simulink model "Cooperative_Localization_05_New"  (R2016b)
settings: Solver=ode45  StartTime=0.0  StopTime=200  RelTol=1e-3  EnableMultiTasking=on
InitFcn:
  | Const_Coop_Local_05
values from neighbouring files (symbols this model uses):
  k1 = 1    [Const_05.m]
  k2 = 1    [Const_05.m]
undefined symbols (not defined in the file or in its folder): alpha, AN, B, B_pseudo_inverse, BBT_inv, BN, D, Delta_form, Gama0, gamma0, gamma_0, gamma_1, H, K, KI, Ki_1, Ki_2, Ki_3, Ki_4, lambda, m_cont, Mb, Mu, n, N, n_cont, Observer_Gain, P_struct, Q, Q1, R, Rho1, Rho_0, rho_0, rho_1, t_cont, U_dot0_M
(part 2 of 3)

== system Cooperative_Localization_05_New/Agent-2/Cooperative controller-2/Decenteralized Cooperaive Controller #2/Estimator A#2/Estimation Error ==
  X : Inport
  U : Inport  Port=2
  G_hat : Inport  Port=3
  Constant : Constant  Value=B
  Constant1 : Constant  Value=D
  Product : Product  Multiplication=Matrix(*)
  Product1 : Product  Multiplication=Matrix(*)
  Scope{1..5} (5 alike) : Scope
  Subsystem : Subsystem
  Subsystem1 : Subsystem
  Subsystem2 : Subsystem
  Subsystem3 : Subsystem
  Sum : Sum  Inputs=+--
  r : Outport
  wt : Outport  Port=2
  wires:
  G_hat/1 -> Product1/2
  Subsystem3/1(X_f) -> r/1, Scope4/1
  X/1 -> Subsystem/1(X), Subsystem3/1(X)
  Subsystem2/1(G_hatf) -> Sum/3, Scope2/1
  Subsystem1/1(Uf) -> Scope1/1, Sum/2
  Subsystem/1(Xf) -> Sum/1, Scope5/1
  Product1/1 -> Subsystem2/1(G_hat)
  Product/1 -> Subsystem1/1(U)
  Constant1/1 -> Product1/1
  U/1 -> Product/2
  Constant/1 -> Product/1
  Sum/1 -> wt/1, Scope3/1

== system Cooperative_Localization_05_New/Agent-2/Cooperative controller-2/Decenteralized Cooperaive Controller #2/Estimator A#2/For matrix Plot1 ==
  A : Inport
  MATLAB Function : MATLAB Function  TreatAsAtomicUnit=on
  To Workspace : ToWorkspace  VariableName=A_hat_2  SaveFormat=Structure With Time  SampleTime=-1
  wires:
  MATLAB Function/1(y) -> To Workspace/1
  A/1 -> MATLAB Function/1(u)

== system Cooperative_Localization_05_New/Agent-2/Cooperative controller-2/Decenteralized Cooperaive Controller #2/Estimator A#2/For matrix Plot2 ==
  A_dot : Inport
  MATLAB Function : MATLAB Function  TreatAsAtomicUnit=on
  To Workspace : ToWorkspace  VariableName=DA_hat_2  SaveFormat=Structure With Time  SampleTime=-1
  wires:
  A_dot/1 -> MATLAB Function/1(u)
  MATLAB Function/1(y) -> To Workspace/1

== system Cooperative_Localization_05_New/Agent-3/Cooperative controller-3/Decenteralized Cooperaive Controller #3/Estimator A#3/Estimation Error ==
  X : Inport
  U : Inport  Port=2
  G_hat : Inport  Port=3
  Constant : Constant  Value=B
  Constant1 : Constant  Value=D
  Product : Product  Multiplication=Matrix(*)
  Product1 : Product  Multiplication=Matrix(*)
  Scope{1..5} (5 alike) : Scope
  Subsystem : Subsystem
  Subsystem1 : Subsystem
  Subsystem2 : Subsystem
  Subsystem3 : Subsystem
  Sum : Sum  Inputs=+--
  r : Outport
  wt : Outport  Port=2
  wires:
  G_hat/1 -> Product1/2
  Subsystem3/1(X_f) -> r/1, Scope4/1
  X/1 -> Subsystem/1(X), Subsystem3/1(X)
  Subsystem2/1(G_hatf) -> Sum/3, Scope2/1
  Subsystem1/1(Uf) -> Scope1/1, Sum/2
  Subsystem/1(Xf) -> Sum/1, Scope5/1
  Product1/1 -> Subsystem2/1(G_hat)
  Product/1 -> Subsystem1/1(U)
  Constant1/1 -> Product1/1
  U/1 -> Product/2
  Constant/1 -> Product/1
  Sum/1 -> wt/1, Scope3/1

== system Cooperative_Localization_05_New/Agent-3/Cooperative controller-3/Decenteralized Cooperaive Controller #3/Estimator A#3/For matrix Plot1 ==
  A : Inport
  MATLAB Function : MATLAB Function  TreatAsAtomicUnit=on
  To Workspace : ToWorkspace  VariableName=A_hat_3  SaveFormat=Structure With Time  SampleTime=-1
  wires:
  MATLAB Function/1(y) -> To Workspace/1
  A/1 -> MATLAB Function/1(u)

== system Cooperative_Localization_05_New/Agent-3/Cooperative controller-3/Decenteralized Cooperaive Controller #3/Estimator A#3/For matrix Plot2 ==
  A_dot : Inport
  MATLAB Function : MATLAB Function  TreatAsAtomicUnit=on
  To Workspace : ToWorkspace  VariableName=DA_hat_3  SaveFormat=Structure With Time  SampleTime=-1
  wires:
  A_dot/1 -> MATLAB Function/1(u)
  MATLAB Function/1(y) -> To Workspace/1

== system Cooperative_Localization_05_New/Agent-4/Cooperative controller-4/Decenteralized Cooperaive Controller #4/Estimator A#4/Estimation Error ==
  X : Inport
  U : Inport  Port=2
  G_hat : Inport  Port=3
  Constant : Constant  Value=B
  Constant1 : Constant  Value=D
  Product : Product  Multiplication=Matrix(*)
  Product1 : Product  Multiplication=Matrix(*)
  Scope{1..5} (5 alike) : Scope
  Subsystem : Subsystem
  Subsystem1 : Subsystem
  Subsystem2 : Subsystem
  Subsystem3 : Subsystem
  Sum : Sum  Inputs=+--
  r : Outport
  wt : Outport  Port=2
  wires:
  G_hat/1 -> Product1/2
  Subsystem3/1(X_f) -> r/1, Scope4/1
  X/1 -> Subsystem/1(X), Subsystem3/1(X)
  Subsystem2/1(G_hatf) -> Sum/3, Scope2/1
  Subsystem1/1(Uf) -> Scope1/1, Sum/2
  Subsystem/1(Xf) -> Sum/1, Scope5/1
  Product1/1 -> Subsystem2/1(G_hat)
  Product/1 -> Subsystem1/1(U)
  Constant1/1 -> Product1/1
  U/1 -> Product/2
  Constant/1 -> Product/1
  Sum/1 -> wt/1, Scope3/1

== system Cooperative_Localization_05_New/Agent-4/Cooperative controller-4/Decenteralized Cooperaive Controller #4/Estimator A#4/For matrix Plot1 ==
  A : Inport
  MATLAB Function : MATLAB Function  TreatAsAtomicUnit=on
  To Workspace : ToWorkspace  VariableName=A_hat_4  SaveFormat=Structure With Time  SampleTime=-1
  wires:
  MATLAB Function/1(y) -> To Workspace/1
  A/1 -> MATLAB Function/1(u)

== system Cooperative_Localization_05_New/Agent-4/Cooperative controller-4/Decenteralized Cooperaive Controller #4/Estimator A#4/For matrix Plot2 ==
  A_dot : Inport
  MATLAB Function : MATLAB Function  TreatAsAtomicUnit=on
  To Workspace : ToWorkspace  VariableName=DA_hat_4  SaveFormat=Structure With Time  SampleTime=-1
  wires:
  A_dot/1 -> MATLAB Function/1(u)
  MATLAB Function/1(y) -> To Workspace/1

== system Cooperative_Localization_05_New/Agent-1/Cooperative controller-1/Decenteralized Cooperaive Controller #1/Estimator A#1/Estimation Error/Subsystem ==
  X : Inport
  Demux : Demux
  Mux : Mux
  Transfer Fcn{,1..3} (4 alike) : TransferFcn  Numerator=[1 0]  Denominator=[1 1]
  Xf : Outport
  wires:
  Demux/1 -> Transfer Fcn/1
  Transfer Fcn/1 -> Mux/1
  Mux/1 -> Xf/1
  X/1 -> Demux/1
  Demux/2 -> Transfer Fcn1/1
  Transfer Fcn1/1 -> Mux/2
  Demux/3 -> Transfer Fcn2/1
  Transfer Fcn2/1 -> Mux/3
  Transfer Fcn3/1 -> Mux/4
  Demux/4 -> Transfer Fcn3/1

== system Cooperative_Localization_05_New/Agent-1/Cooperative controller-1/Decenteralized Cooperaive Controller #1/Estimator A#1/Estimation Error/Subsystem1 ==
  U : Inport
  Demux : Demux
  Mux : Mux
  Transfer Fcn{1..4} (4 alike) : TransferFcn  Denominator=[1 1]
  Uf : Outport
  wires:
  U/1 -> Demux/1
  Mux/1 -> Uf/1
  Transfer Fcn1/1 -> Mux/1
  Demux/1 -> Transfer Fcn1/1
  Transfer Fcn2/1 -> Mux/2
  Demux/2 -> Transfer Fcn2/1
  Demux/3 -> Transfer Fcn3/1
  Transfer Fcn3/1 -> Mux/3
  Transfer Fcn4/1 -> Mux/4
  Demux/4 -> Transfer Fcn4/1

== system Cooperative_Localization_05_New/Agent-1/Cooperative controller-1/Decenteralized Cooperaive Controller #1/Estimator A#1/Estimation Error/Subsystem2 ==
  G_hat : Inport
  Demux : Demux
  Mux : Mux
  Transfer Fcn{1..4} (4 alike) : TransferFcn  Denominator=[1 1]
  G_hatf : Outport
  wires:
  Demux/1 -> Transfer Fcn2/1
  Transfer Fcn2/1 -> Mux/1
  Mux/1 -> G_hatf/1
  G_hat/1 -> Demux/1
  Demux/2 -> Transfer Fcn1/1
  Transfer Fcn1/1 -> Mux/2
  Demux/3 -> Transfer Fcn3/1
  Transfer Fcn3/1 -> Mux/3
  Demux/4 -> Transfer Fcn4/1
  Transfer Fcn4/1 -> Mux/4

== system Cooperative_Localization_05_New/Agent-1/Cooperative controller-1/Decenteralized Cooperaive Controller #1/Estimator A#1/Estimation Error/Subsystem3 ==
  X : Inport
  Demux : Demux
  Mux : Mux
  Transfer Fcn{1..4} (4 alike) : TransferFcn  Denominator=[1 1]
  X_f : Outport
  wires:
  X/1 -> Demux/1
  Mux/1 -> X_f/1
  Transfer Fcn2/1 -> Mux/1
  Demux/1 -> Transfer Fcn2/1
  Demux/2 -> Transfer Fcn1/1
  Transfer Fcn1/1 -> Mux/2
  Demux/3 -> Transfer Fcn3/1
  Transfer Fcn3/1 -> Mux/3
  Demux/4 -> Transfer Fcn4/1
  Transfer Fcn4/1 -> Mux/4

== system Cooperative_Localization_05_New/Agent-2/Cooperative controller-2/Decenteralized Cooperaive Controller #2/Estimator A#2/Estimation Error/Subsystem ==
  X : Inport
  Demux : Demux
  Mux : Mux
  Transfer Fcn{,1..3} (4 alike) : TransferFcn  Numerator=[1 0]  Denominator=[1 1]
  Xf : Outport
  wires:
  Demux/1 -> Transfer Fcn/1
  Transfer Fcn/1 -> Mux/1
  Mux/1 -> Xf/1
  X/1 -> Demux/1
  Demux/2 -> Transfer Fcn1/1
  Transfer Fcn1/1 -> Mux/2
  Demux/3 -> Transfer Fcn2/1
  Transfer Fcn2/1 -> Mux/3
  Transfer Fcn3/1 -> Mux/4
  Demux/4 -> Transfer Fcn3/1

== system Cooperative_Localization_05_New/Agent-2/Cooperative controller-2/Decenteralized Cooperaive Controller #2/Estimator A#2/Estimation Error/Subsystem1 ==
  U : Inport
  Demux : Demux
  Mux : Mux
  Transfer Fcn{1..4} (4 alike) : TransferFcn  Denominator=[1 1]
  Uf : Outport
  wires:
  U/1 -> Demux/1
  Mux/1 -> Uf/1
  Transfer Fcn1/1 -> Mux/1
  Demux/1 -> Transfer Fcn1/1
  Transfer Fcn2/1 -> Mux/2
  Demux/2 -> Transfer Fcn2/1
  Demux/3 -> Transfer Fcn3/1
  Transfer Fcn3/1 -> Mux/3
  Transfer Fcn4/1 -> Mux/4
  Demux/4 -> Transfer Fcn4/1

== system Cooperative_Localization_05_New/Agent-2/Cooperative controller-2/Decenteralized Cooperaive Controller #2/Estimator A#2/Estimation Error/Subsystem2 ==
  G_hat : Inport
  Demux : Demux
  Mux : Mux
  Transfer Fcn{1..4} (4 alike) : TransferFcn  Denominator=[1 1]
  G_hatf : Outport
  wires:
  Demux/1 -> Transfer Fcn2/1
  Transfer Fcn2/1 -> Mux/1
  Mux/1 -> G_hatf/1
  G_hat/1 -> Demux/1
  Demux/2 -> Transfer Fcn1/1
  Transfer Fcn1/1 -> Mux/2
  Demux/3 -> Transfer Fcn3/1
  Transfer Fcn3/1 -> Mux/3
  Demux/4 -> Transfer Fcn4/1
  Transfer Fcn4/1 -> Mux/4

== system Cooperative_Localization_05_New/Agent-2/Cooperative controller-2/Decenteralized Cooperaive Controller #2/Estimator A#2/Estimation Error/Subsystem3 ==
  X : Inport
  Demux : Demux
  Mux : Mux
  Transfer Fcn{1..4} (4 alike) : TransferFcn  Denominator=[1 1]
  X_f : Outport
  wires:
  X/1 -> Demux/1
  Mux/1 -> X_f/1
  Transfer Fcn2/1 -> Mux/1
  Demux/1 -> Transfer Fcn2/1
  Demux/2 -> Transfer Fcn1/1
  Transfer Fcn1/1 -> Mux/2
  Demux/3 -> Transfer Fcn3/1
  Transfer Fcn3/1 -> Mux/3
  Demux/4 -> Transfer Fcn4/1
  Transfer Fcn4/1 -> Mux/4

== system Cooperative_Localization_05_New/Agent-3/Cooperative controller-3/Decenteralized Cooperaive Controller #3/Estimator A#3/Estimation Error/Subsystem ==
  X : Inport
  Demux : Demux
  Mux : Mux
  Transfer Fcn{,1..3} (4 alike) : TransferFcn  Numerator=[1 0]  Denominator=[1 1]
  Xf : Outport
  wires:
  Demux/1 -> Transfer Fcn/1
  Transfer Fcn/1 -> Mux/1
  Mux/1 -> Xf/1
  X/1 -> Demux/1
  Demux/2 -> Transfer Fcn1/1
  Transfer Fcn1/1 -> Mux/2
  Demux/3 -> Transfer Fcn2/1
  Transfer Fcn2/1 -> Mux/3
  Transfer Fcn3/1 -> Mux/4
  Demux/4 -> Transfer Fcn3/1

== system Cooperative_Localization_05_New/Agent-3/Cooperative controller-3/Decenteralized Cooperaive Controller #3/Estimator A#3/Estimation Error/Subsystem1 ==
  U : Inport
  Demux : Demux
  Mux : Mux
  Transfer Fcn{1..4} (4 alike) : TransferFcn  Denominator=[1 1]
  Uf : Outport
  wires:
  U/1 -> Demux/1
  Mux/1 -> Uf/1
  Transfer Fcn1/1 -> Mux/1
  Demux/1 -> Transfer Fcn1/1
  Transfer Fcn2/1 -> Mux/2
  Demux/2 -> Transfer Fcn2/1
  Demux/3 -> Transfer Fcn3/1
  Transfer Fcn3/1 -> Mux/3
  Transfer Fcn4/1 -> Mux/4
  Demux/4 -> Transfer Fcn4/1

== system Cooperative_Localization_05_New/Agent-3/Cooperative controller-3/Decenteralized Cooperaive Controller #3/Estimator A#3/Estimation Error/Subsystem2 ==
  G_hat : Inport
  Demux : Demux
  Mux : Mux
  Transfer Fcn{1..4} (4 alike) : TransferFcn  Denominator=[1 1]
  G_hatf : Outport
  wires:
  Demux/1 -> Transfer Fcn2/1
  Transfer Fcn2/1 -> Mux/1
  Mux/1 -> G_hatf/1
  G_hat/1 -> Demux/1
  Demux/2 -> Transfer Fcn1/1
  Transfer Fcn1/1 -> Mux/2
  Demux/3 -> Transfer Fcn3/1
  Transfer Fcn3/1 -> Mux/3
  Demux/4 -> Transfer Fcn4/1
  Transfer Fcn4/1 -> Mux/4

== system Cooperative_Localization_05_New/Agent-3/Cooperative controller-3/Decenteralized Cooperaive Controller #3/Estimator A#3/Estimation Error/Subsystem3 ==
  X : Inport
  Demux : Demux
  Mux : Mux
  Transfer Fcn{1..4} (4 alike) : TransferFcn  Denominator=[1 1]
  X_f : Outport
  wires:
  X/1 -> Demux/1
  Mux/1 -> X_f/1
  Transfer Fcn2/1 -> Mux/1
  Demux/1 -> Transfer Fcn2/1
  Demux/2 -> Transfer Fcn1/1
  Transfer Fcn1/1 -> Mux/2
  Demux/3 -> Transfer Fcn3/1
  Transfer Fcn3/1 -> Mux/3
  Demux/4 -> Transfer Fcn4/1
  Transfer Fcn4/1 -> Mux/4

== system Cooperative_Localization_05_New/Agent-4/Cooperative controller-4/Decenteralized Cooperaive Controller #4/Estimator A#4/Estimation Error/Subsystem ==
  X : Inport
  Demux : Demux
  Mux : Mux
  Transfer Fcn{,1..3} (4 alike) : TransferFcn  Numerator=[1 0]  Denominator=[1 1]
  Xf : Outport
  wires:
  Demux/1 -> Transfer Fcn/1
  Transfer Fcn/1 -> Mux/1
  Mux/1 -> Xf/1
  X/1 -> Demux/1
  Demux/2 -> Transfer Fcn1/1
  Transfer Fcn1/1 -> Mux/2
  Demux/3 -> Transfer Fcn2/1
  Transfer Fcn2/1 -> Mux/3
  Transfer Fcn3/1 -> Mux/4
  Demux/4 -> Transfer Fcn3/1

== system Cooperative_Localization_05_New/Agent-4/Cooperative controller-4/Decenteralized Cooperaive Controller #4/Estimator A#4/Estimation Error/Subsystem1 ==
  U : Inport
  Demux : Demux
  Mux : Mux
  Transfer Fcn{1..4} (4 alike) : TransferFcn  Denominator=[1 1]
  Uf : Outport
  wires:
  U/1 -> Demux/1
  Mux/1 -> Uf/1
  Transfer Fcn1/1 -> Mux/1
  Demux/1 -> Transfer Fcn1/1
  Transfer Fcn2/1 -> Mux/2
  Demux/2 -> Transfer Fcn2/1
  Demux/3 -> Transfer Fcn3/1
  Transfer Fcn3/1 -> Mux/3
  Transfer Fcn4/1 -> Mux/4
  Demux/4 -> Transfer Fcn4/1

== system Cooperative_Localization_05_New/Agent-4/Cooperative controller-4/Decenteralized Cooperaive Controller #4/Estimator A#4/Estimation Error/Subsystem2 ==
  G_hat : Inport
  Demux : Demux
  Mux : Mux
  Transfer Fcn{1..4} (4 alike) : TransferFcn  Denominator=[1 1]
  G_hatf : Outport
  wires:
  Demux/1 -> Transfer Fcn2/1
  Transfer Fcn2/1 -> Mux/1
  Mux/1 -> G_hatf/1
  G_hat/1 -> Demux/1
  Demux/2 -> Transfer Fcn1/1
  Transfer Fcn1/1 -> Mux/2
  Demux/3 -> Transfer Fcn3/1
  Transfer Fcn3/1 -> Mux/3
  Demux/4 -> Transfer Fcn4/1
  Transfer Fcn4/1 -> Mux/4

== system Cooperative_Localization_05_New/Agent-4/Cooperative controller-4/Decenteralized Cooperaive Controller #4/Estimator A#4/Estimation Error/Subsystem3 ==
  X : Inport
  Demux : Demux
  Mux : Mux
  Transfer Fcn{1..4} (4 alike) : TransferFcn  Denominator=[1 1]
  X_f : Outport
  wires:
  X/1 -> Demux/1
  Mux/1 -> X_f/1
  Transfer Fcn2/1 -> Mux/1
  Demux/1 -> Transfer Fcn2/1
  Demux/2 -> Transfer Fcn1/1
  Transfer Fcn1/1 -> Mux/2
  Demux/3 -> Transfer Fcn3/1
  Transfer Fcn3/1 -> Mux/3
  Demux/4 -> Transfer Fcn4/1
  Transfer Fcn4/1 -> Mux/4

== matlab function Cooperative_Localization_05_New/Agent-1/Cooperative controller-1/Choosing real control variables ==
  data: u output; U input
function u = fcn(U)

u = U(3:4);

end

== matlab function Cooperative_Localization_05_New/Agent-1/Agent-1/MATLAB Function ==
  data: Px input; Py input; Vx input; out output; Vy input; Ax input; Ay input; t input
function out = fcn(Px,Py,Vx,Vy,Ax,Ay,t)

DPx = Vx;
DPy = Vy;

DVx = Ax - Vx * sin(0.2*t) + 0.5 * Px * cos(0.1*t);
DVy = Ay - Vy * sin(0.2*t) + 0.5 * Py * cos(0.1*t);

out = [DPx;DPy;DVx;DVy];

end

== matlab function Cooperative_Localization_05_New/Agent-2/Agent-2/MATLAB Function ==
  data: Px input; Py input; Vx input; out output; Vy input; Ax input; Ay input; t input
function out = fcn(Px,Py,Vx,Vy,Ax,Ay,t)

DPx = Vx;
DPy = Vy;

DVx = Ax - Vx * sin(0.2*t) + 0.5 * Px * cos(0.1*t);
DVy = Ay - Vy * sin(0.2*t) + 0.5 * Py * cos(0.1*t);

out = [DPx;DPy;DVx;DVy];

end

== matlab function Cooperative_Localization_05_New/Agent-2/Relative positions-2/Relative estimation ==
  data: V_rel input; d input; DP_est output; P_est input; alpha parameter
function DP_est = fcn(V_rel,d,P_est,alpha)

e = (d^2) - (P_est'*P_est);
g = P_est'*V_rel;

DP_est = (1 + alpha * sign(e*g)) * V_rel;

end

== matlab function Cooperative_Localization_05_New/Agent-2/Relative positions-2/Relative estimation1 ==
  data: V_rel input; d input; DP_est output; P_est input; alpha parameter
function DP_est = fcn(V_rel,d,P_est,alpha)

e = (d^2) - (P_est'*P_est);
g = P_est'*V_rel;

DP_est = (1 + alpha * sign(e*g)) * V_rel;

end

== matlab function Cooperative_Localization_05_New/Agent-2/Relative positions-2/Relative estimation2 ==
  data: V_rel input; d input; DP_est output; P_est input; alpha parameter
function DP_est = fcn(V_rel,d,P_est,alpha)

e = (d^2) - (P_est'*P_est);
g = P_est'*V_rel;

DP_est = (1 + alpha * sign(e*g)) * V_rel;

end

== matlab function Cooperative_Localization_05_New/Agent-2/Relative positions-2/Relative estimation3 ==
  data: V_rel input; d input; DP_est output; P_est input; alpha parameter
function DP_est = fcn(V_rel,d,P_est,alpha)

e = (d^2) - (P_est'*P_est);
g = P_est'*V_rel;

DP_est = (1 + alpha * sign(e*g)) * V_rel;

end

== matlab function Cooperative_Localization_05_New/Agent-1/observer-1 ==
  data: P_hat input; tau input; P0 input; P_rel_local input; P_rel0_local input; AN parameter; BN parameter; H parameter; DP_hat_local output; n parameter; N parameter; Num input; Mu parameter; Mb parameter; tau_i output; alpha parameter
function [DP_hat_local,tau_i] = fcn(P_hat,tau,P0,P_rel_local,P_rel0_local,AN,BN,H,n,N,Num,Mu,Mb,alpha)

P_hat_in = zeros(n,N);
P_rel_local_in = zeros(n,N);
tau_in = zeros(n,N);
for i=1:N
    P_hat_in(:,i) = P_hat((i-1)*n+1:(i*n),1); 
    P_rel_local_in(:,i) = P_rel_local((i-1)*n+1:(i*n),1); 
    tau_in(:,i) = tau((i-1)*n+1:(i*n),1);
end

e = BN(Num,Num)*(P_hat_in(:,Num) - (P0 + P_rel0_local));
Vec = zeros(n,1);
for i=1:N
    e = e + ( AN(Num,i)*(P_hat_in(:,Num) - (P_hat_in(:,i) + P_rel_local_in(:,i))) ); 
    Vec = Vec + ( H(Num,i)*tau_in(:,i) );    
end

SGN_vec = Vec./(abs(Vec)+alpha);
SGN = diag(SGN_vec);    

DP_hat_local = - ( Mu*e ) - ( SGN*Mb );
tau_i = e;

end

== matlab function Cooperative_Localization_05_New/Agent-3/Relative positions-3/Relative estimation ==
  data: V_rel input; d input; DP_est output; P_est input; alpha parameter
function DP_est = fcn(V_rel,d,P_est,alpha)

e = (d^2) - (P_est'*P_est);
g = P_est'*V_rel;

DP_est = (1 + alpha * sign(e*g)) * V_rel;

end

== matlab function Cooperative_Localization_05_New/Agent-1/Relative positions-1/Relative estimation2 ==
  data: V_rel input; d input; DP_est output; P_est input; alpha parameter
function DP_est = fcn(V_rel,d,P_est,alpha)

e = (d^2) - (P_est'*P_est);
g = P_est'*V_rel;

DP_est = (1 + alpha * sign(e*g)) * V_rel;

end

== matlab function Cooperative_Localization_05_New/Agent-3/Relative positions-3/Relative estimation2 ==
  data: V_rel input; d input; DP_est output; P_est input; alpha parameter
function DP_est = fcn(V_rel,d,P_est,alpha)

e = (d^2) - (P_est'*P_est);
g = P_est'*V_rel;

DP_est = (1 + alpha * sign(e*g)) * V_rel;

end

== matlab function Cooperative_Localization_05_New/Agent-3/Relative positions-3/Relative estimation1 ==
  data: V_rel input; d input; DP_est output; P_est input; alpha parameter
function DP_est = fcn(V_rel,d,P_est,alpha)

e = (d^2) - (P_est'*P_est);
g = P_est'*V_rel;

DP_est = (1 + alpha * sign(e*g)) * V_rel;

end

== matlab function Cooperative_Localization_05_New/Agent-3/Relative positions-3/Relative estimation3 ==
  data: V_rel input; d input; DP_est output; P_est input; alpha parameter
function DP_est = fcn(V_rel,d,P_est,alpha)

e = (d^2) - (P_est'*P_est);
g = P_est'*V_rel;

DP_est = (1 + alpha * sign(e*g)) * V_rel;

end

== matlab function Cooperative_Localization_05_New/Agent-1/Cooperative controller-1/Decenteralized Cooperaive Controller #1/Adaptive Law #1 ==
  data: Agent_Num input; G_hat input; Gama0 parameter; P input; P_struct parameter; DG_hat output; E input; H parameter; D parameter; N parameter; n_cont parameter; t_cont parameter; Rho_0 parameter
function DG_hat = fcn(Agent_Num,G_hat,Gama0,P,P_struct,E,H,D,N,n_cont,t_cont,Rho_0)

P_struct(1).data = P.p1;
P_struct(2).data = P.p2;
P_struct(3).data = P.p3;
P_struct(4).data = P.p4;

Sum = zeros(t_cont,1);
for i=1:N  
    Sum = Sum + (H(i,Agent_Num) * D' * P_struct(i).data * E((i-1)*n_cont+1:(i*n_cont),1)); %Adaptive law
end

DG_hat = +( Gama0*Sum - (Rho_0*Gama0*G_hat) );
    
end

== matlab function Cooperative_Localization_05_New/Agent-1/Relative positions-1/Relative estimation1 ==
  data: V_rel input; d input; DP_est output; P_est input; alpha parameter
function DP_est = fcn(V_rel,d,P_est,alpha)

e = (d^2) - (P_est'*P_est);
g = P_est'*V_rel;

DP_est = (1 + alpha * sign(e*g)) * V_rel;

end

== matlab function Cooperative_Localization_05_New/Agent-1/Relative positions-1/Relative estimation3 ==
  data: V_rel input; d input; DP_est output; P_est input; alpha parameter
function DP_est = fcn(V_rel,d,P_est,alpha)

e = (d^2) - (P_est'*P_est);
g = P_est'*V_rel;

DP_est = (1 + alpha * sign(e*g)) * V_rel;

end

== matlab function Cooperative_Localization_05_New/Agent-1/Relative positions-1/Relative estimation ==
  data: V_rel input; d input; DP_est output; P_est input; alpha parameter
function DP_est = fcn(V_rel,d,P_est,alpha)

e = (d^2) - (P_est'*P_est);
g = P_est'*V_rel;

DP_est = (1 + alpha * sign(e*g)) * V_rel;

end

== matlab function Cooperative_Localization_05_New/Agent-1/Relative positions-1/Relative measurements ==
  data: P1 input; d output; P2 input
function d = fcn(P1,P2)

d = sqrt( (P2(1) - P1(1))^2 + (P2(2) - P1(2))^2 );

end

== matlab function Cooperative_Localization_05_New/Agent-4/Relative positions-4/Relative estimation ==
  data: V_rel input; d input; DP_est output; P_est input; alpha parameter
function DP_est = fcn(V_rel,d,P_est,alpha)

e = (d^2) - (P_est'*P_est);
g = P_est'*V_rel;

DP_est = (1 + alpha * sign(e*g)) * V_rel;

end

== matlab function Cooperative_Localization_05_New/Agent-4/Relative positions-4/Relative estimation1 ==
  data: V_rel input; d input; DP_est output; P_est input; alpha parameter
function DP_est = fcn(V_rel,d,P_est,alpha)

e = (d^2) - (P_est'*P_est);
g = P_est'*V_rel;

DP_est = (1 + alpha * sign(e*g)) * V_rel;

end

== matlab function Cooperative_Localization_05_New/Agent-4/Relative positions-4/Relative estimation2 ==
  data: V_rel input; d input; DP_est output; P_est input; alpha parameter
function DP_est = fcn(V_rel,d,P_est,alpha)

e = (d^2) - (P_est'*P_est);
g = P_est'*V_rel;

DP_est = (1 + alpha * sign(e*g)) * V_rel;

end

== matlab function Cooperative_Localization_05_New/Agent-1/Relative positions-1/Relative measurements1 ==
  data: P1 input; d output; P2 input
function d = fcn(P1,P2)

d = sqrt( (P2(1) - P1(1))^2 + (P2(2) - P1(2))^2 );

end

== matlab function Cooperative_Localization_05_New/Agent-4/Relative positions-4/Relative estimation3 ==
  data: V_rel input; d input; DP_est output; P_est input; alpha parameter
function DP_est = fcn(V_rel,d,P_est,alpha)

e = (d^2) - (P_est'*P_est);
g = P_est'*V_rel;

DP_est = (1 + alpha * sign(e*g)) * V_rel;

end

== matlab function Cooperative_Localization_05_New/Agent-3/Agent-3/MATLAB Function ==
  data: Px input; Py input; Vx input; out output; Vy input; Ax input; Ay input; t input
function out = fcn(Px,Py,Vx,Vy,Ax,Ay,t)

DPx = Vx;
DPy = Vy;

DVx = Ax - Vx * sin(0.2*t) + 0.5 * Px * cos(0.1*t);
DVy = Ay - Vy * sin(0.2*t) + 0.5 * Py * cos(0.1*t);

out = [DPx;DPy;DVx;DVy];

end

== matlab function Cooperative_Localization_05_New/Agent-4/Agent-4/MATLAB Function ==
  data: Px input; Py input; Vx input; out output; Vy input; Ax input; Ay input; t input
function out = fcn(Px,Py,Vx,Vy,Ax,Ay,t)

DPx = Vx;
DPy = Vy;

DVx = Ax - Vx * sin(0.2*t) + 0.5 * Px * cos(0.1*t);
DVy = Ay - Vy * sin(0.2*t) + 0.5 * Py * cos(0.1*t);

out = [DPx;DPy;DVx;DVy];

end

== matlab function Cooperative_Localization_05_New/Agent-1/Relative positions-1/Relative measurements2 ==
  data: P1 input; d output; P2 input
function d = fcn(P1,P2)

d = sqrt( (P2(1) - P1(1))^2 + (P2(2) - P1(2))^2 );

end

== matlab function Cooperative_Localization_05_New/Leader/Agent-0/MATLAB Function ==
  data: Px input; Py input; Vx input; out output; Vy input; Ax input; Ay input; t input
function out = fcn(Px,Py,Vx,Vy,Ax,Ay,t)

DPx = Vx;
DPy = Vy;

DVx = Ax - Vx * sin(0.2*t) + 0.5 * Px * cos(0.1*t);
DVy = Ay - Vy * sin(0.2*t) + 0.5 * Py * cos(0.1*t);

out = [DPx;DPy;DVx;DVy];

end

== matlab function Cooperative_Localization_05_New/Agent-1/Relative positions-1/Relative measurements3 ==
  data: P1 input; d output; P2 input
function d = fcn(P1,P2)

d = sqrt( (P2(1) - P1(1))^2 + (P2(2) - P1(2))^2 );

end

== matlab function Cooperative_Localization_05_New/Agent-2/Relative positions-2/Relative measurements ==
  data: P1 input; d output; P2 input
function d = fcn(P1,P2)

d = sqrt( (P2(1) - P1(1))^2 + (P2(2) - P1(2))^2 );

end

== matlab function Cooperative_Localization_05_New/Agent-2/Relative positions-2/Relative measurements1 ==
  data: P1 input; d output; P2 input
function d = fcn(P1,P2)

d = sqrt( (P2(1) - P1(1))^2 + (P2(2) - P1(2))^2 );

end

== matlab function Cooperative_Localization_05_New/Agent-2/Relative positions-2/Relative measurements2 ==
  data: P1 input; d output; P2 input
function d = fcn(P1,P2)

d = sqrt( (P2(1) - P1(1))^2 + (P2(2) - P1(2))^2 );

end

== matlab function Cooperative_Localization_05_New/Agent-2/Relative positions-2/Relative measurements3 ==
  data: P1 input; d output; P2 input
function d = fcn(P1,P2)

d = sqrt( (P2(1) - P1(1))^2 + (P2(2) - P1(2))^2 );

end

== matlab function Cooperative_Localization_05_New/Agent-2/Cooperative controller-2/Choosing real control variables ==
  data: u output; U input
function u = fcn(U)

u = U(3:4);

end

== matlab function Cooperative_Localization_05_New/Agent-2/Cooperative controller-2/Decenteralized Cooperaive Controller #2/Adaptive Law #2 ==
  data: Agent_Num input; G_hat input; Gama0 parameter; P input; P_struct parameter; DG_hat output; E input; H parameter; D parameter; N parameter; n_cont parameter; t_cont parameter; Rho_0 parameter
function DG_hat = fcn(Agent_Num,G_hat,Gama0,P,P_struct,E,H,D,N,n_cont,t_cont,Rho_0)

P_struct(1).data = P.p1;
P_struct(2).data = P.p2;
P_struct(3).data = P.p3;
P_struct(4).data = P.p4;

Sum = zeros(t_cont,1);
for i=1:N  
    Sum = Sum + (H(i,Agent_Num) * D' * P_struct(i).data * E((i-1)*n_cont+1:(i*n_cont),1)); %Adaptive law
end

DG_hat = +( Gama0*Sum - (Rho_0*Gama0*G_hat) );
    
end

== matlab function Cooperative_Localization_05_New/Agent-2/observer-1 ==
  data: P_hat input; tau input; P0 input; P_rel_local input; P_rel0_local input; AN parameter; BN parameter; H parameter; DP_hat_local output; n parameter; N parameter; Num input; Mu parameter; Mb parameter; tau_i output; alpha parameter
function [DP_hat_local,tau_i] = fcn(P_hat,tau,P0,P_rel_local,P_rel0_local,AN,BN,H,n,N,Num,Mu,Mb,alpha)

P_hat_in = zeros(n,N);
P_rel_local_in = zeros(n,N);
tau_in = zeros(n,N);
for i=1:N
    P_hat_in(:,i) = P_hat((i-1)*n+1:(i*n),1); 
    P_rel_local_in(:,i) = P_rel_local((i-1)*n+1:(i*n),1); 
    tau_in(:,i) = tau((i-1)*n+1:(i*n),1);
end

e = BN(Num,Num)*(P_hat_in(:,Num) - (P0 + P_rel0_local));
Vec = zeros(n,1);
for i=1:N
    e = e + ( AN(Num,i)*(P_hat_in(:,Num) - (P_hat_in(:,i) + P_rel_local_in(:,i))) ); 
    Vec = Vec + ( H(Num,i)*tau_in(:,i) );    
end

SGN_vec = Vec./(abs(Vec)+alpha);
SGN = diag(SGN_vec);    

DP_hat_local = - ( Mu*e ) - ( SGN*Mb );
tau_i = e;

end

== matlab function Cooperative_Localization_05_New/Agent-3/Relative positions-3/Relative measurements ==
  data: P1 input; d output; P2 input
function d = fcn(P1,P2)

d = sqrt( (P2(1) - P1(1))^2 + (P2(2) - P1(2))^2 );

end

== matlab function Cooperative_Localization_05_New/Agent-3/Relative positions-3/Relative measurements1 ==
  data: P1 input; d output; P2 input
function d = fcn(P1,P2)

d = sqrt( (P2(1) - P1(1))^2 + (P2(2) - P1(2))^2 );

end

== matlab function Cooperative_Localization_05_New/Agent-3/Relative positions-3/Relative measurements2 ==
  data: P1 input; d output; P2 input
function d = fcn(P1,P2)

d = sqrt( (P2(1) - P1(1))^2 + (P2(2) - P1(2))^2 );

end

== matlab function Cooperative_Localization_05_New/Agent-3/Relative positions-3/Relative measurements3 ==
  data: P1 input; d output; P2 input
function d = fcn(P1,P2)

d = sqrt( (P2(1) - P1(1))^2 + (P2(2) - P1(2))^2 );

end

== matlab function Cooperative_Localization_05_New/Agent-3/Cooperative controller-3/Choosing real control variables ==
  data: u output; U input
function u = fcn(U)

u = U(3:4);

end

== matlab function Cooperative_Localization_05_New/Agent-3/Cooperative controller-3/Decenteralized Cooperaive Controller #3/Adaptive Law #3 ==
  data: Agent_Num input; G_hat input; Gama0 parameter; P input; P_struct parameter; DG_hat output; E input; H parameter; D parameter; N parameter; n_cont parameter; t_cont parameter; Rho_0 parameter
function DG_hat = fcn(Agent_Num,G_hat,Gama0,P,P_struct,E,H,D,N,n_cont,t_cont,Rho_0)

P_struct(1).data = P.p1;
P_struct(2).data = P.p2;
P_struct(3).data = P.p3;
P_struct(4).data = P.p4;

Sum = zeros(t_cont,1);
for i=1:N  
    Sum = Sum + (H(i,Agent_Num) * D' * P_struct(i).data * E((i-1)*n_cont+1:(i*n_cont),1)); %Adaptive law
end

DG_hat = +( Gama0*Sum - (Rho_0*Gama0*G_hat) );
    
end

== matlab function Cooperative_Localization_05_New/Agent-3/observer-1 ==
  data: P_hat input; tau input; P0 input; P_rel_local input; P_rel0_local input; AN parameter; BN parameter; H parameter; DP_hat_local output; n parameter; N parameter; Num input; Mu parameter; Mb parameter; tau_i output; alpha parameter
function [DP_hat_local,tau_i] = fcn(P_hat,tau,P0,P_rel_local,P_rel0_local,AN,BN,H,n,N,Num,Mu,Mb,alpha)

P_hat_in = zeros(n,N);
P_rel_local_in = zeros(n,N);
tau_in = zeros(n,N);
for i=1:N
    P_hat_in(:,i) = P_hat((i-1)*n+1:(i*n),1); 
    P_rel_local_in(:,i) = P_rel_local((i-1)*n+1:(i*n),1); 
    tau_in(:,i) = tau((i-1)*n+1:(i*n),1);
end

e = BN(Num,Num)*(P_hat_in(:,Num) - (P0 + P_rel0_local));
Vec = zeros(n,1);
for i=1:N
    e = e + ( AN(Num,i)*(P_hat_in(:,Num) - (P_hat_in(:,i) + P_rel_local_in(:,i))) ); 
    Vec = Vec + ( H(Num,i)*tau_in(:,i) );    
end

SGN_vec = Vec./(abs(Vec)+alpha);
SGN = diag(SGN_vec);    

DP_hat_local = - ( Mu*e ) - ( SGN*Mb );
tau_i = e;

end

== matlab function Cooperative_Localization_05_New/Agent-4/Cooperative controller-4/Choosing real control variables ==
  data: u output; U input
function u = fcn(U)

u = U(3:4);

end

== matlab function Cooperative_Localization_05_New/Agent-4/Relative positions-4/Relative measurements ==
  data: P1 input; d output; P2 input
function d = fcn(P1,P2)

d = sqrt( (P2(1) - P1(1))^2 + (P2(2) - P1(2))^2 );

end

== matlab function Cooperative_Localization_05_New/Agent-4/Relative positions-4/Relative measurements1 ==
  data: P1 input; d output; P2 input
function d = fcn(P1,P2)

d = sqrt( (P2(1) - P1(1))^2 + (P2(2) - P1(2))^2 );

end

== matlab function Cooperative_Localization_05_New/Agent-4/Relative positions-4/Relative measurements2 ==
  data: P1 input; d output; P2 input
function d = fcn(P1,P2)

d = sqrt( (P2(1) - P1(1))^2 + (P2(2) - P1(2))^2 );

end

== matlab function Cooperative_Localization_05_New/Agent-4/Relative positions-4/Relative measurements3 ==
  data: P1 input; d output; P2 input
function d = fcn(P1,P2)

d = sqrt( (P2(1) - P1(1))^2 + (P2(2) - P1(2))^2 );

end

== matlab function Cooperative_Localization_05_New/Agent-4/Cooperative controller-4/Decenteralized Cooperaive Controller #4/Adaptive Law #4 ==
  data: Agent_Num input; G_hat input; Gama0 parameter; P input; P_struct parameter; DG_hat output; E input; H parameter; D parameter; N parameter; n_cont parameter; t_cont parameter; Rho_0 parameter
function DG_hat = fcn(Agent_Num,G_hat,Gama0,P,P_struct,E,H,D,N,n_cont,t_cont,Rho_0)

P_struct(1).data = P.p1;
P_struct(2).data = P.p2;
P_struct(3).data = P.p3;
P_struct(4).data = P.p4;

Sum = zeros(t_cont,1);
for i=1:N  
    Sum = Sum + (H(i,Agent_Num) * D' * P_struct(i).data * E((i-1)*n_cont+1:(i*n_cont),1)); %Adaptive law
end

DG_hat = +( Gama0*Sum - (Rho_0*Gama0*G_hat) );
    
end

== matlab function Cooperative_Localization_05_New/Agent-1/Cooperative controller-1/Decenteralized Cooperaive Controller #1/Approx. U#1 ==
  data: T_i input; Approx_U_i output; B_pseudo_inverse parameter; A_i input; X_i input; D parameter; G_hat_i input
function Approx_U_i  = fcn(T_i,B_pseudo_inverse,A_i,X_i,D,G_hat_i)

Approx_U_i = B_pseudo_inverse * (T_i - A_i * X_i + D * G_hat_i);

end

== matlab function Cooperative_Localization_05_New/Agent-4/observer-1 ==
  data: P_hat input; tau input; P0 input; P_rel_local input; P_rel0_local input; AN parameter; BN parameter; H parameter; DP_hat_local output; n parameter; N parameter; Num input; Mu parameter; Mb parameter; tau_i output; alpha parameter
function [DP_hat_local,tau_i] = fcn(P_hat,tau,P0,P_rel_local,P_rel0_local,AN,BN,H,n,N,Num,Mu,Mb,alpha)

P_hat_in = zeros(n,N);
P_rel_local_in = zeros(n,N);
tau_in = zeros(n,N);
for i=1:N
    P_hat_in(:,i) = P_hat((i-1)*n+1:(i*n),1); 
    P_rel_local_in(:,i) = P_rel_local((i-1)*n+1:(i*n),1); 
    tau_in(:,i) = tau((i-1)*n+1:(i*n),1);
end

e = BN(Num,Num)*(P_hat_in(:,Num) - (P0 + P_rel0_local));
Vec = zeros(n,1);
for i=1:N
    e = e + ( AN(Num,i)*(P_hat_in(:,Num) - (P_hat_in(:,i) + P_rel_local_in(:,i))) ); 
    Vec = Vec + ( H(Num,i)*tau_in(:,i) );    
end

SGN_vec = Vec./(abs(Vec)+alpha);
SGN = diag(SGN_vec);    

DP_hat_local = - ( Mu*e ) - ( SGN*Mb );
tau_i = e;

end

== matlab function Cooperative_Localization_05_New/Agent-1/Cooperative controller-1/Decenteralized Cooperaive Controller #1/Estimator A#1/For matrix Plot1/MATLAB Function ==
  data: u input; y output
function y = fcn(u)
S1 = size(u,1);
S2 = size(u,2);

y = zeros(S1*S2,1);
num = 0;
for i=1:S1
    for j=1:S2
        num = num + 1;
        y(num,1) = u(i,j);
    end
end

end

== matlab function Cooperative_Localization_05_New/Agent-1/Cooperative controller-1/Decenteralized Cooperaive Controller #1/Estimator A#1/For matrix Plot2/MATLAB Function ==
  data: u input; y output
function y = fcn(u)
S1 = size(u,1);
S2 = size(u,2);

y = zeros(S1*S2,1);
num = 0;
for i=1:S1
    for j=1:S2
        num = num + 1;
        y(num,1) = u(i,j);
    end
end

end

== matlab function Cooperative_Localization_05_New/Agent-1/Cooperative controller-1/Decenteralized Cooperaive Controller #1/Estimator A#1/parameter online identification ==
  data: r input; DA_hat output; Wt input; lambda parameter; A_hat input; Rho1 parameter; n_cont parameter
function DA_hat = fcn(r,Wt,lambda,A_hat,Rho1,n_cont)

eps = (Wt - A_hat*r)/(1+0.001);

DA_hat = (lambda * eps * r') - (Rho1 * lambda * A_hat); 

end

== matlab function Cooperative_Localization_05_New/Agent-1/Cooperative controller-1/Decenteralized Cooperaive Controller #1/For matrix Plot/MATLAB Function ==
  data: u input; y output
function y = fcn(u)
S1 = size(u,1);
S2 = size(u,2);

y = zeros(S1*S2,1);
num = 0;
for i=1:S1
    for j=1:S2
        num = num + 1;
        y(num,1) = u(i,j);
    end
end

end

== matlab function Cooperative_Localization_05_New/Agent-1/Cooperative controller-1/Decenteralized Cooperaive Controller #1/Main Controller #1 ==
  data: n_cont parameter; U output; K parameter; P_i input; E_i input; KI parameter; Zeta_i input; BN parameter; A_i input; U_0 input; Z_0 input; N parameter; H parameter; D parameter; B parameter; G_hat input; t_cont parameter; Delta_form parameter; m_cont parameter; Approx_U input; Agent_Num input; B_pseudo_inverse parameter
function U = fcn(n_cont,K,P_i,E_i,KI,Zeta_i,BN,A_i,U_0,Z_0,N,H,D,B,G_hat,t_cont,Delta_form,m_cont,Approx_U,Agent_Num,B_pseudo_inverse)

K_i = K((Agent_Num-1)*n_cont+1:(Agent_Num*n_cont),(Agent_Num-1)*n_cont+1:(Agent_Num*n_cont));
U1 = - K_i * P_i * E_i; %Consensus Error

KI_i = KI((Agent_Num-1)*n_cont+1:(Agent_Num*n_cont),(Agent_Num-1)*n_cont+1:(Agent_Num*n_cont));
U2 = - KI_i * Zeta_i; %Consensus time-integral

U3 = + BN(Agent_Num,Agent_Num)*(U_0-A_i*Z_0); %Connection to the leader

U4 = zeros(n_cont,1);
U5 = zeros(n_cont,1);
U6 = zeros(n_cont,1);
for i=1:N
    U4 = U4 - (H(Agent_Num,i)*A_i*Delta_form(:,i)); %Formation parameters
    
    U5 = U5 - (H(Agent_Num,i)*D*G_hat((i-1)*t_cont+1:(i*t_cont),1)); %Adaptive part
    
    if i~= Agent_Num
        U6 = U6 - (H(Agent_Num,i)*B*Approx_U((i-1)*m_cont+1:(i*m_cont),1)); %Observer on leader
    end
end

U_input = U1 + U2 + U3 + U4 + U5 + U6;

U = B_pseudo_inverse * U_input / H(Agent_Num,Agent_Num);

end

== matlab function Cooperative_Localization_05_New/Agent-1/Cooperative controller-1/Decenteralized Cooperaive Controller #1/Observer #1 ==
  data: T input; DT_i output; Delta input; H parameter; BN parameter; AN parameter; T_i input; U0 input; U_dot0_M parameter; Delta_i output; N parameter; n_cont parameter; Agent_Num input; Observer_Gain parameter
function [DT_i,Delta_i] = fcn(T,Delta,H,BN,AN,T_i,U0,U_dot0_M,N,n_cont,Agent_Num,Observer_Gain)

Delta_i = + BN(Agent_Num,Agent_Num)*(T_i - U0);
Sum2 = zeros(n_cont,1);
for i=1:N
    Delta_i = Delta_i + ( AN(Agent_Num,i) * (T_i - T(((i-1)*n_cont+1):n_cont*i)) );  
    Sum2 = Sum2 + ( H(i,Agent_Num) * Delta(((i-1)*n_cont+1):n_cont*i) );
end

Sum21 = abs(Sum2) + 0.01*ones(n_cont,1);
SGN2 = Sum2./Sum21;

DT_i = -Observer_Gain*Delta_i - diag(SGN2)*U_dot0_M;

end

== matlab function Cooperative_Localization_05_New/Agent-1/Cooperative controller-1/Decenteralized Cooperaive Controller #1/Riccati equation ==
  data: A_hat input; K_i input; Q parameter; P_i output; gamma0 parameter; n_cont parameter
function P_i = care_sol(A_hat,K_i,Q,gamma0,n_cont)

% Reference: "Numerical Solution of Algebraic Riccati Equations" by: "Dario A. Bini" - Page 194 in PDF.
% CARE: A'X + XA - XBX = -C
% gamma should be negative EX. = -1;

A = A_hat + 1e-3*eye(n_cont);
B = K_i;
C = Q;
gamma = gamma0;

tol = 1e-13;
kmax = 30;

Ai = inv(A+(gamma*eye(n_cont)));
R = B*Ai'*C;
S1 = inv(A+(gamma*eye(n_cont))+R);
E = S1*(A-(gamma*eye(n_cont))+R);
R = eye(n_cont)-(Ai*(A-(gamma*eye(n_cont))));
G = S1*B*R';
P = -S1'*C*R;

err = 1;
ki = 0;

while err>tol && ki<kmax
    IGP = eye(n_cont) - G*P;
    Z = [E;P']/IGP;
    E1 = Z(1:n_cont,:);
    P1 = Z(n_cont+1:end,:);
    G = G + (E1*G*E');
    P = P + (E'*P1'*E);
    E = E1*E;
    err = norm(E,1);
    ki = ki+1;
end

P_i = P;

end

== matlab function Cooperative_Localization_05_New/Agent-1/Cooperative controller-1/Module to compute Consensus Error #1 ==
  data: P_rel_all input; P_rel0 input; V_loc input; V0 input; V_all input; Ep output; AN parameter; BN parameter; Delta_form parameter; N parameter; n_cont parameter; Agent_Num input; n parameter
function Ep = fcn(P_rel_all,P_rel0,V_loc,V0,V_all,AN,BN,Delta_form,N,n_cont,Agent_Num, n)

Diff_Star_to0 = Delta_form(:,Agent_Num); 
Diff_Star_to_Other = ( eye(n_cont) * Diff_Star_to0 * ones(1,N) ) - Delta_form;

%% ---------------------------------------------------------------

Ep = ( BN(Agent_Num,Agent_Num)*([P_rel0;(V_loc-V0)]-Diff_Star_to0) ); 

for i=1:N        
    Ep = Ep + AN(Agent_Num,i)*([P_rel_all((n*(i-1)+1):(i*n),1);(V_loc-V_all((n*(i-1)+1):(i*n),1))]-Diff_Star_to_Other(:,i));
end

end

== matlab function Cooperative_Localization_05_New/Agent-1/Cooperative controller-1/Variable change ==
  data: U input; X input; X_mod output; n_cont parameter
function X_mod = fcn(U,X,n_cont)

X_mod = zeros(n_cont,1);
X_mod(1:2) = X(1:2);
X_mod(3:4) = X(3:4) - U(1:2);

end

== matlab function Cooperative_Localization_05_New/Agent-2/Cooperative controller-2/Module to compute Consensus Error #2 ==
  data: P_rel_all input; P_rel0 input; V_loc input; V0 input; V_all input; Ep output; AN parameter; BN parameter; Delta_form parameter; N parameter; n_cont parameter; Agent_Num input; n parameter
function Ep = fcn(P_rel_all,P_rel0,V_loc,V0,V_all,AN,BN,Delta_form,N,n_cont,Agent_Num, n)

Diff_Star_to0 = Delta_form(:,Agent_Num); 
Diff_Star_to_Other = ( eye(n_cont) * Diff_Star_to0 * ones(1,N) ) - Delta_form;

%% ---------------------------------------------------------------

Ep = ( BN(Agent_Num,Agent_Num)*([P_rel0;(V_loc-V0)]-Diff_Star_to0) );

for i=1:N        
    Ep = Ep + AN(Agent_Num,i)*([P_rel_all((n*(i-1)+1):(i*n),1);(V_loc-V_all((n*(i-1)+1):(i*n),1))]-Diff_Star_to_Other(:,i));
end

end

== matlab function Cooperative_Localization_05_New/Agent-2/Cooperative controller-2/Decenteralized Cooperaive Controller #2/Approx. U#2 ==
  data: T_i input; Approx_U_i output; B_pseudo_inverse parameter; A_i input; X_i input; D parameter; G_hat_i input
function Approx_U_i  = fcn(T_i,B_pseudo_inverse,A_i,X_i,D,G_hat_i)

Approx_U_i = B_pseudo_inverse * (T_i - A_i * X_i + D * G_hat_i);

end

== matlab function Cooperative_Localization_05_New/Agent-2/Cooperative controller-2/Decenteralized Cooperaive Controller #2/Estimator A#2/For matrix Plot1/MATLAB Function ==
  data: u input; y output
function y = fcn(u)
S1 = size(u,1);
S2 = size(u,2);

y = zeros(S1*S2,1);
num = 0;
for i=1:S1
    for j=1:S2
        num = num + 1;
        y(num,1) = u(i,j);
    end
end

end

== matlab function Cooperative_Localization_05_New/Agent-2/Cooperative controller-2/Decenteralized Cooperaive Controller #2/Estimator A#2/For matrix Plot2/MATLAB Function ==
  data: u input; y output
function y = fcn(u)
S1 = size(u,1);
S2 = size(u,2);

y = zeros(S1*S2,1);
num = 0;
for i=1:S1
    for j=1:S2
        num = num + 1;
        y(num,1) = u(i,j);
    end
end

end

== matlab function Cooperative_Localization_05_New/Agent-2/Cooperative controller-2/Decenteralized Cooperaive Controller #2/Estimator A#2/parameter online identification ==
  data: r input; DA_hat output; Wt input; lambda parameter; A_hat input; Rho1 parameter; n_cont parameter
function DA_hat = fcn(r,Wt,lambda,A_hat,Rho1,n_cont)

eps = (Wt - A_hat*r)/(1+0.001);

DA_hat = (lambda * eps * r') - (Rho1 * lambda * A_hat); 

end

== matlab function Cooperative_Localization_05_New/Agent-2/Cooperative controller-2/Decenteralized Cooperaive Controller #2/For matrix Plot/MATLAB Function ==
  data: u input; y output
function y = fcn(u)
S1 = size(u,1);
S2 = size(u,2);

y = zeros(S1*S2,1);
num = 0;
for i=1:S1
    for j=1:S2
        num = num + 1;
        y(num,1) = u(i,j);
    end
end

end

== matlab function Cooperative_Localization_05_New/Agent-2/Cooperative controller-2/Decenteralized Cooperaive Controller #2/Main Controller #2 ==
  data: n_cont parameter; U output; K parameter; P_i input; E_i input; KI parameter; Zeta_i input; BN parameter; A_i input; U_0 input; Z_0 input; N parameter; H parameter; D parameter; B parameter; G_hat input; t_cont parameter; Delta_form parameter; m_cont parameter; Approx_U input; Agent_Num input; B_pseudo_inverse parameter
function U = fcn(n_cont,K,P_i,E_i,KI,Zeta_i,BN,A_i,U_0,Z_0,N,H,D,B,G_hat,t_cont,Delta_form,m_cont,Approx_U,Agent_Num,B_pseudo_inverse)

K_i = K((Agent_Num-1)*n_cont+1:(Agent_Num*n_cont),(Agent_Num-1)*n_cont+1:(Agent_Num*n_cont));
U1 = - K_i * P_i * E_i; %Consensus Error

KI_i = KI((Agent_Num-1)*n_cont+1:(Agent_Num*n_cont),(Agent_Num-1)*n_cont+1:(Agent_Num*n_cont));
U2 = - KI_i * Zeta_i; %Consensus time-integral

U3 = + BN(Agent_Num,Agent_Num)*(U_0-A_i*Z_0); %Connection to the leader

U4 = zeros(n_cont,1);
U5 = zeros(n_cont,1);
U6 = zeros(n_cont,1);
for i=1:N
    U4 = U4 - (H(Agent_Num,i)*A_i*Delta_form(:,i)); %Formation parameters
    
    U5 = U5 - (H(Agent_Num,i)*D*G_hat((i-1)*t_cont+1:(i*t_cont),1)); %Adaptive part
    
    if i~= Agent_Num
        U6 = U6 - (H(Agent_Num,i)*B*Approx_U((i-1)*m_cont+1:(i*m_cont),1)); %Observer on leader
    end
end

U_input = U1 + U2 + U3 + U4 + U5 + U6;

U = B_pseudo_inverse * U_input / H(Agent_Num,Agent_Num);

end

== matlab function Cooperative_Localization_05_New/Agent-2/Cooperative controller-2/Decenteralized Cooperaive Controller #2/Observer #2 ==
  data: T input; DT_i output; Delta input; H parameter; BN parameter; AN parameter; T_i input; U0 input; U_dot0_M parameter; Delta_i output; N parameter; n_cont parameter; Agent_Num input; Observer_Gain parameter
function [DT_i,Delta_i] = fcn(T,Delta,H,BN,AN,T_i,U0,U_dot0_M,N,n_cont,Agent_Num,Observer_Gain)

Delta_i = + BN(Agent_Num,Agent_Num)*(T_i - U0);
Sum2 = zeros(n_cont,1);
for i=1:N
    Delta_i = Delta_i + ( AN(Agent_Num,i) * (T_i - T(((i-1)*n_cont+1):n_cont*i)) );  
    Sum2 = Sum2 + ( H(i,Agent_Num) * Delta(((i-1)*n_cont+1):n_cont*i) );
end

Sum21 = abs(Sum2) + 0.01*ones(n_cont,1);
SGN2 = Sum2./Sum21;

DT_i = -Observer_Gain*Delta_i - diag(SGN2)*U_dot0_M;

end

== matlab function Cooperative_Localization_05_New/Agent-2/Cooperative controller-2/Decenteralized Cooperaive Controller #2/Riccati equation ==
  data: A_hat input; K_i input; Q parameter; P_i output; gamma0 parameter; n_cont parameter
function P_i = care_sol(A_hat,K_i,Q,gamma0,n_cont)

% Reference: "Numerical Solution of Algebraic Riccati Equations" by: "Dario A. Bini" - Page 194 in PDF.
% CARE: A'X + XA - XBX = -C
% gamma should be negative EX. = -1;

A = A_hat + 1e-3*eye(n_cont);
B = K_i;
C = Q;
gamma = gamma0;

tol = 1e-13;
kmax = 30;

Ai = inv(A+(gamma*eye(n_cont)));
R = B*Ai'*C;
S1 = inv(A+(gamma*eye(n_cont))+R);
E = S1*(A-(gamma*eye(n_cont))+R);
R = eye(n_cont)-(Ai*(A-(gamma*eye(n_cont))));
G = S1*B*R';
P = -S1'*C*R;

err = 1;
ki = 0;

while err>tol && ki<kmax
    IGP = eye(n_cont) - G*P;
    Z = [E;P']/IGP;
    E1 = Z(1:n_cont,:);
    P1 = Z(n_cont+1:end,:);
    G = G + (E1*G*E');
    P = P + (E'*P1'*E);
    E = E1*E;
    err = norm(E,1);
    ki = ki+1;
end

P_i = P;

end

== matlab function Cooperative_Localization_05_New/Agent-3/Cooperative controller-3/Module to compute Consensus Error #3 ==
  data: P_rel_all input; P_rel0 input; V_loc input; V0 input; V_all input; Ep output; AN parameter; BN parameter; Delta_form parameter; N parameter; n_cont parameter; Agent_Num input; n parameter
function Ep = fcn(P_rel_all,P_rel0,V_loc,V0,V_all,AN,BN,Delta_form,N,n_cont,Agent_Num, n)

Diff_Star_to0 = Delta_form(:,Agent_Num); 
Diff_Star_to_Other = ( eye(n_cont) * Diff_Star_to0 * ones(1,N) ) - Delta_form;

%% ---------------------------------------------------------------

Ep = ( BN(Agent_Num,Agent_Num)*([P_rel0;(V_loc-V0)]-Diff_Star_to0) );

for i=1:N        
    Ep = Ep + AN(Agent_Num,i)*([P_rel_all((n*(i-1)+1):(i*n),1);(V_loc-V_all((n*(i-1)+1):(i*n),1))]-Diff_Star_to_Other(:,i));
end

end

== matlab function Cooperative_Localization_05_New/Agent-2/Cooperative controller-2/Variable change ==
  data: U input; X input; X_mod output; n_cont parameter
function X_mod = fcn(U,X,n_cont)

X_mod = zeros(n_cont,1);
X_mod(1:2) = X(1:2);
X_mod(3:4) = X(3:4) - U(1:2);

end

== matlab function Cooperative_Localization_05_New/Agent-3/Cooperative controller-3/Decenteralized Cooperaive Controller #3/Approx. U#3 ==
  data: T_i input; Approx_U_i output; B_pseudo_inverse parameter; A_i input; X_i input; D parameter; G_hat_i input
function Approx_U_i  = fcn(T_i,B_pseudo_inverse,A_i,X_i,D,G_hat_i)

Approx_U_i = B_pseudo_inverse * (T_i - A_i * X_i + D * G_hat_i);

end

== matlab function Cooperative_Localization_05_New/Agent-3/Cooperative controller-3/Decenteralized Cooperaive Controller #3/Estimator A#3/For matrix Plot1/MATLAB Function ==
  data: u input; y output
function y = fcn(u)
S1 = size(u,1);
S2 = size(u,2);

y = zeros(S1*S2,1);
num = 0;
for i=1:S1
    for j=1:S2
        num = num + 1;
        y(num,1) = u(i,j);
    end
end

end

== matlab function Cooperative_Localization_05_New/Agent-3/Cooperative controller-3/Decenteralized Cooperaive Controller #3/Estimator A#3/For matrix Plot2/MATLAB Function ==
  data: u input; y output
function y = fcn(u)
S1 = size(u,1);
S2 = size(u,2);

y = zeros(S1*S2,1);
num = 0;
for i=1:S1
    for j=1:S2
        num = num + 1;
        y(num,1) = u(i,j);
    end
end

end

== matlab function Cooperative_Localization_05_New/Agent-3/Cooperative controller-3/Decenteralized Cooperaive Controller #3/Estimator A#3/parameter online identification ==
  data: r input; DA_hat output; Wt input; lambda parameter; A_hat input; Rho1 parameter; n_cont parameter
function DA_hat = fcn(r,Wt,lambda,A_hat,Rho1,n_cont)

eps = (Wt - A_hat*r)/(1+0.001);

DA_hat = (lambda * eps * r') - (Rho1 * lambda * A_hat); 

end

== matlab function Cooperative_Localization_05_New/Agent-3/Cooperative controller-3/Decenteralized Cooperaive Controller #3/For matrix Plot/MATLAB Function ==
  data: u input; y output
function y = fcn(u)
S1 = size(u,1);
S2 = size(u,2);

y = zeros(S1*S2,1);
num = 0;
for i=1:S1
    for j=1:S2
        num = num + 1;
        y(num,1) = u(i,j);
    end
end

end

== matlab function Cooperative_Localization_05_New/Agent-3/Cooperative controller-3/Decenteralized Cooperaive Controller #3/Main Controller #3 ==
  data: n_cont parameter; U output; K parameter; P_i input; E_i input; KI parameter; Zeta_i input; BN parameter; A_i input; U_0 input; Z_0 input; N parameter; H parameter; D parameter; B parameter; G_hat input; t_cont parameter; Delta_form parameter; m_cont parameter; Approx_U input; Agent_Num input; B_pseudo_inverse parameter
function U = fcn(n_cont,K,P_i,E_i,KI,Zeta_i,BN,A_i,U_0,Z_0,N,H,D,B,G_hat,t_cont,Delta_form,m_cont,Approx_U,Agent_Num,B_pseudo_inverse)

K_i = K((Agent_Num-1)*n_cont+1:(Agent_Num*n_cont),(Agent_Num-1)*n_cont+1:(Agent_Num*n_cont));
U1 = - K_i * P_i * E_i; %Consensus Error

KI_i = KI((Agent_Num-1)*n_cont+1:(Agent_Num*n_cont),(Agent_Num-1)*n_cont+1:(Agent_Num*n_cont));
U2 = - KI_i * Zeta_i; %Consensus time-integral

U3 = + BN(Agent_Num,Agent_Num)*(U_0-A_i*Z_0); %Connection to the leader

U4 = zeros(n_cont,1);
U5 = zeros(n_cont,1);
U6 = zeros(n_cont,1);
for i=1:N
    U4 = U4 - (H(Agent_Num,i)*A_i*Delta_form(:,i)); %Formation parameters
    
    U5 = U5 - (H(Agent_Num,i)*D*G_hat((i-1)*t_cont+1:(i*t_cont),1)); %Adaptive part
    
    if i~= Agent_Num
        U6 = U6 - (H(Agent_Num,i)*B*Approx_U((i-1)*m_cont+1:(i*m_cont),1)); %Observer on leader
    end
end

U_input = U1 + U2 + U3 + U4 + U5 + U6;

U = B_pseudo_inverse * U_input / H(Agent_Num,Agent_Num);

end
